simulink model "varianza_tiempo"  (R2023b)
settings: Solver=VariableStepAuto  StartTime=0.0  StopTime=10.0  RelTol=1e-3
settings Model: Creator=luisG  LastModifiedBy=diavl
settings OptimizationCC: ReuseModelBlockBuffer=off

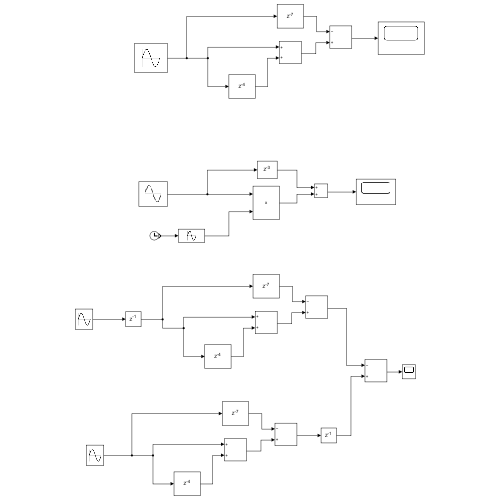
[thumbnail: Simulink's stored preview of the top-level diagram]
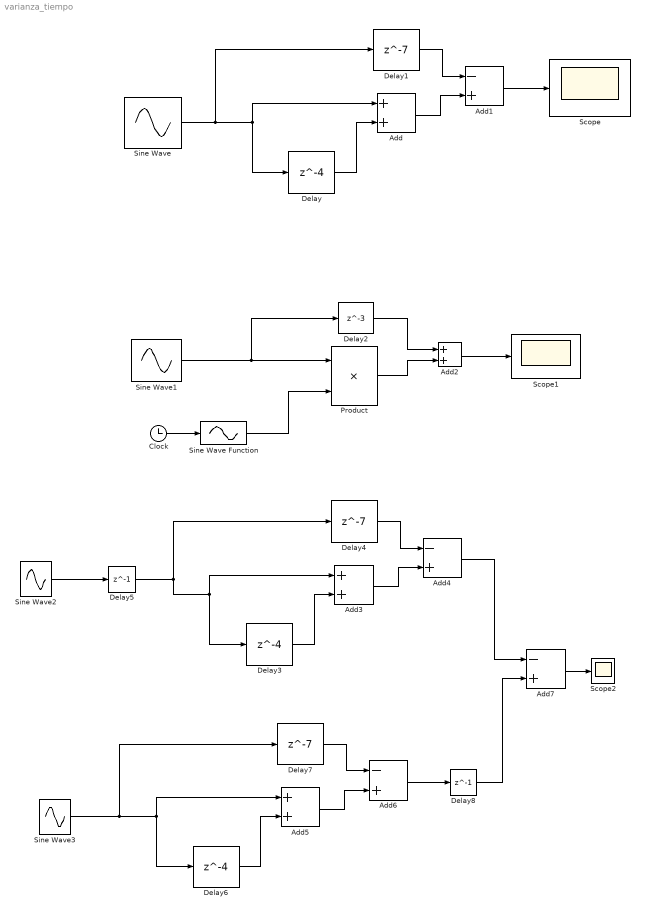
== system varianza_tiempo ==
  Add{,2..3,5} (4 alike) : Sum
  Add{1,4,6..7} (4 alike) : Sum  Inputs=-+
  Clock : Clock
  Delay : Delay  DelayLength=4  InitialCondition=0
  Delay1 : Delay  DelayLength=7  InitialCondition=0
  Delay2 : Delay  DelayLength=3  InitialCondition=0
  Delay3 : Delay  DelayLength=4  InitialCondition=0
  Delay4 : Delay  DelayLength=7  InitialCondition=0
  Delay5 : Delay  DelayLength=1  InitialCondition=0
  Delay6 : Delay  DelayLength=4  InitialCondition=0
  Delay7 : Delay  DelayLength=7  InitialCondition=0
  Delay8 : Delay  DelayLength=1  InitialCondition=0
  Product : Product
  Scope : Scope
  Scope1 : Scope
  Scope2 : Scope
  Sine Wave{,1..3} (4 alike) : Sin  SampleTime=0
  Sine Wave Function : Sin  TimeSource=Use external signal  SampleTime=0
  wires:
  Sine Wave/1 -> Delay1/1, Add/1, Delay/1
  Delay/1 -> Add/2
  Delay1/1 -> Add1/1
  Add/1 -> Add1/2
  Sine Wave1/1 -> Delay2/1, Product/1
  Clock/1 -> Sine Wave Function/1
  Sine Wave Function/1 -> Product/2
  Delay2/1 -> Add2/1
  Product/1 -> Add2/2
  Add2/1 -> Scope1/1
  Add1/1 -> Scope/1
  Add3/1 -> Add4/2
  Delay5/1 -> Add3/1, Delay3/1, Delay4/1
  Delay3/1 -> Add3/2
  Delay4/1 -> Add4/1
  Sine Wave2/1 -> Delay5/1
  Add5/1 -> Add6/2
  Sine Wave3/1 -> Delay7/1, Add5/1, Delay6/1
  Delay6/1 -> Add5/2
  Delay7/1 -> Add6/1
  Add6/1 -> Delay8/1
  Add4/1 -> Add7/1
  Delay8/1 -> Add7/2
  Add7/1 -> Scope2/1
